simulink model "Part2"  (R2024b)
settings: Solver=ode4  StartTime=0.0  StopTime=T_SIM  FixedStep=T_s  RelTol=1e-3
values from neighbouring files (symbols this model uses):
  D = diag([0.001, 0.001, 0.0175/6, 0.0175/6, 0.0175/6, 0.0175/6*T_s, 0.0175/6*T_s].^2)    [P2_script.m]    (also in workspace_full.mat = [1e-06 0 0 0 0 0 0 0 1e-06 0 0 0 ... (49 elements, 7x7)])
  d_id = d_cal_hat    [P2_script.m]
  H = [H_motion_cap ; H_enc; H_gyro]    [P2_script.m]    (also in workspace_full.mat = [0 0 0 0 0 0 1 0 0 1 0 0 ... (14 elements, 2x7)])
  H_enc = [0, 0, 0, 1, 0, 0, 0 ... (first row only)    [P2_script.m]
  H_gyro = [0, 0, 0, 0, 0, -r_id/d_id, r_id/d_id]    [P2_script.m]
  H_motion_cap = [1, 0, 0, 0, 0, 0, 0 ... (first row only)    [P2_script.m]
  P_INIT_EKF = diag([0.001, 0.001, 0.0175/6, 0.0175/6, 0.0175/6, 0.0175/6*T_s, 0.0175/6*T_s].^2)    [P2_script.m]    (also in workspace_full.mat = [1e-06 0 0 0 0 0 0 0 1e-06 0 0 0 ... (49 elements, 7x7)])
  p_loss = p_loss_values(3)    [P2_script.m]
  PHI_INIT = [0;0]    [P2_script.m]    (also in workspace_full.mat = [0 0])
  Q_INIT_LOC = Q_INIT    [P2_script.m]    (also in workspace_full.mat = [0 0 0.463647609001])
  R_1 = diag([ENCODER_QUANTIZATION/6, ENCODER_QUANTIZATION/6].^2)    [P2_script.m]
  R_2 = diag(([ENCODER_QUANTIZATION/6, ENCODER_QUANTIZATION/6, var_IMU]).^2)    [P2_script.m]    (also in workspace_full.mat = [6.53638071556e-08  0; 0  6.53638071556e-08])
  R_3 = diag(([var_motion_capture, var_motion_capture, var_motion_capture,               ENCODER_QUANTIZATION/6, ENCODER_QUANTIZATION/6, var_IMU]).^2)    [P2_script.m]    (also in workspace_full.mat = [1e-06  0  0; 0  6.53638071556e-08  0; 0  0  6.53638071556e-)
  r_id = r_cal_hat    [P2_script.m]
  T_s = 0.04    [P2_script.m]    (also in workspace_full.mat)
  test_case = 3    [P2_script.m]
  Z_INIT_EKF = [Q_INIT; 0; 0; 0; 0]    [P2_script.m]    (also in workspace_full.mat = [0 0 0.463647609001 0 0 0 0])
settings Model: Creator=tomailoren  LastModifiedBy=loren
settings OptimizationCC: DefaultParameterBehavior=Inlined  EnhancedBackFolding=on  PassReuseOutputArgsAs=Individual arguments  ZeroExternalMemoryAtStartup=off  ZeroInternalMemoryAtStartup=off  MaxStackSize=64  OptimizeBlockOrder=speed  DifferentSizesBufferReuse=on  OptimizationCustomize=off  EfficientTunableParamExpr=on
settings DebuggingCC: ParameterTunabilityLossMsg=error
settings HardwareCC: ProdBitPerPointer=32  ProdBitPerSizeT=32  ProdBitPerPtrDiffT=32  ProdLargestAtomicFloat=None  ProdIntDivRoundTo=Undefined  ProdEndianess=Unspecified  ProdWordSize=32  ProdHWDeviceType=Generic->Unspecified (assume 32-bit Generic)
settings SFSimCC: MATLABDynamicMemAlloc=off
settings RTWCC: Description=Embedded Coder  SystemTargetFile=ert.tlc  HardwareBoard=Robot Operating System (ROS)  TLCOptions="-aInlineSetEventsForThisBaseRateFcn=TLC_FALSE -aSuppressMultiTaskScheduler=TLC_FALSE  -aRateBasedStepFcn=0"  TemplateMakefile=ert_default_tmf  Toolchain=Catkin  TargetLang=C++
settings CodeAppCC: ForceParamTrailComments=on  IgnoreCustomStorageClasses=off  OperatorAnnotations=on  SimulinkDataObjDesc=on  SFDataObjDesc=on  InsertBlockDesc=on

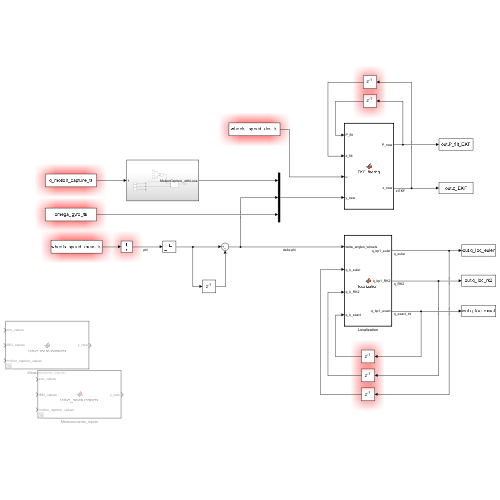
[thumbnail: Simulink's stored preview of the top-level diagram]
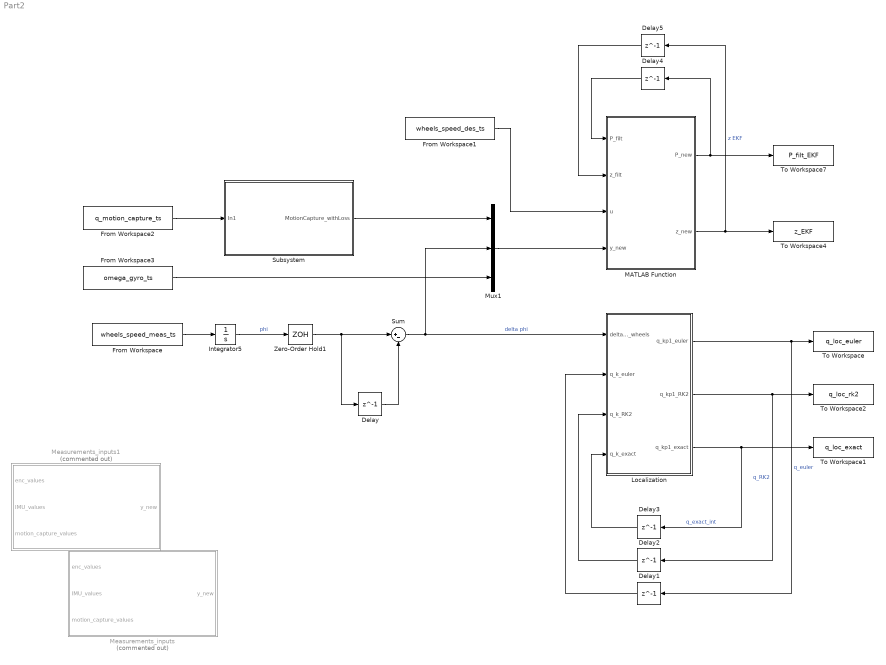
== system Part2 ==
  Delay : Delay  DelayLength=1  InitialCondition=[0;0]  SampleTime=T_s
  Delay1 : Delay  DelayLength=1  InitialCondition=Q_INIT_LOC
  Delay2 : Delay  DelayLength=1  InitialCondition=Q_INIT_LOC
  Delay3 : Delay  DelayLength=1  InitialCondition=Q_INIT_LOC
  Delay4 : Delay  DelayLength=1  InitialCondition=P_INIT_EKF  SampleTime=T_s
  Delay5 : Delay  DelayLength=1  InitialCondition=Z_INIT_EKF  SampleTime=T_s
  From Workspace : FromWorkspace  VariableName=wheels_speed_meas_ts
  From Workspace1 : FromWorkspace  VariableName=wheels_speed_des_ts
  From Workspace2 : FromWorkspace  VariableName=q_motion_capture_ts
  From Workspace3 : FromWorkspace  VariableName=omega_gyro_ts
  Integrator5 : Integrator  InitialCondition=PHI_INIT
  Localization : MATLAB Function  TreatAsAtomicUnit=on
  MATLAB Function : MATLAB Function  TreatAsAtomicUnit=on
  Measurements_inputs : MATLAB Function  Commented=on  TreatAsAtomicUnit=on
  Measurements_inputs1 : MATLAB Function  Commented=on  TreatAsAtomicUnit=on
  Mux1 : Mux  Inputs=3
  Subsystem : Subsystem
  Sum : Sum  Inputs=|+-
  To Workspace : ToWorkspace  VariableName=q_loc_euler  SaveFormat=Structure With Time  SampleTime=-1
  To Workspace1 : ToWorkspace  VariableName=q_loc_exact  SaveFormat=Structure With Time  SampleTime=-1
  To Workspace2 : ToWorkspace  VariableName=q_loc_rk2  SaveFormat=Structure With Time  SampleTime=-1
  To Workspace4 : ToWorkspace  VariableName=z_EKF  SaveFormat=Structure With Time  SampleTime=-1
  To Workspace7 : ToWorkspace  VariableName=P_filt_EKF  SaveFormat=Structure With Time  SampleTime=-1
  Zero-Order Hold1 : ZeroOrderHold  SampleTime=T_s
  wires:
  MATLAB Function/2(z_new) -> Delay5/1, To Workspace4/1  "z EKF"
  Delay1/1 -> Localization/2(q_k_euler)
  Zero-Order Hold1/1 -> Delay/1, Sum/1
  Delay5/1 -> MATLAB Function/2(z_filt)
  Delay/1 -> Sum/2
  Delay3/1 -> Localization/4(q_k_exact)
  Integrator5/1 -> Zero-Order Hold1/1  "phi"
  Localization/2(q_kp1_RK2) -> To Workspace2/1, Delay2/1  "q_RK2"
  Localization/1(q_kp1_euler) -> To Workspace/1, Delay1/1  "q_euler"
  Delay2/1 -> Localization/3(q_k_RK2)
  Sum/1 -> Mux1/2, Localization/1(delta_angles_wheels)  "delta phi"
  Delay4/1 -> MATLAB Function/1(P_filt)
  Localization/3(q_kp1_exact) -> To Workspace1/1, Delay3/1  "q_exact_int"
  MATLAB Function/1(P_new) -> Delay4/1, To Workspace7/1
  From Workspace/1 -> Integrator5/1
  From Workspace1/1 -> MATLAB Function/3(u)
  Mux1/1 -> MATLAB Function/4(y_new)
  From Workspace3/1 -> Mux1/3
  From Workspace2/1 -> Subsystem/1(In1)
  Subsystem/1(MotionCapture_withLoss) -> Mux1/1

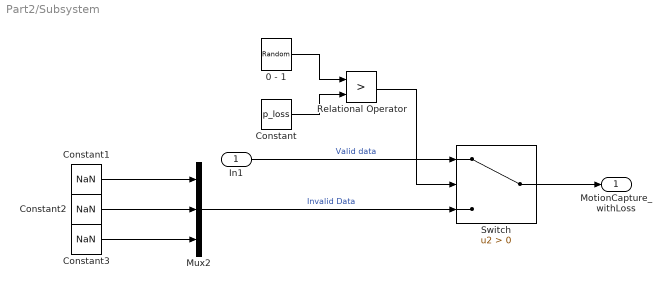
== system Part2/Subsystem ==
  In1 : Inport
  0 - 1 : UniformRandomNumber  Minimum=0  SampleTime=T_s
  Constant : Constant  Value=p_loss
  Constant1 : Constant  Value=NaN
  Constant2 : Constant  Value=NaN
  Constant3 : Constant  Value=NaN
  Mux2 : Mux  Inputs=3
  Relational Operator : RelationalOperator  Operator=>  OutDataTypeStr=boolean  RndMeth=Simplest  InputSameDT=off
  Switch : Switch  Criteria=u2 > Threshold  SaturateOnIntegerOverflow=off  InputSameDT=off
  MotionCapture_withLoss : Outport
  wires:
  0 - 1/1 -> Relational Operator/1
  Constant/1 -> Relational Operator/2
  Switch/1 -> MotionCapture_withLoss/1
  Relational Operator/1 -> Switch/2
  Constant2/1 -> Mux2/2
  Mux2/1 -> Switch/3  "Invalid Data"
  Constant1/1 -> Mux2/1
  In1/1 -> Switch/1  "Valid data"
  Constant3/1 -> Mux2/3

== matlab function Part2/Measurements_inputs1 ==
  data: enc_values input; y_new output; IMU_values input; motion_capture_values input; test_case parameter
function y_new = select_measurements(enc_values, IMU_values, motion_capture_values, test_case)
   
    % enc_values (delta_phi)
    % IMU_values (w_gyro)
    % Motion_capture (state q)

    y_new = zeros(6, 1);
    % y_new = [x; y; theta; delta_phi_L; delta_phi_R; omega_gyro]
    
    if test_case == 1
        % Test 1: Only Encoder
        y_new(4) = enc_values(1);
        y_new(5) = enc_values(2);
        
    elseif test_case == 2
        % Test 2: Encoder + IMU
        y_new(4) = enc_values(1);
        y_new(5) = enc_values(2);
        y_new(6) = IMU_values(1);
        
    elseif test_case == 3
        % Test 3: Encoder + IMU + Motion Capture
        y_new(1) = motion_capture_values(1);
        y_new(2) = motion_capture_values(2);
        y_new(3) = motion_capture_values(3);
        y_new(4) = enc_values(1);
        y_new(5) = enc_values(2);
        y_new(6) = IMU_values(1);
    end
end

== matlab function Part2/Measurements_inputs ==
  data: enc_values input; y_new output; IMU_values input; motion_capture_values input; test_case parameter
function y_new = select_measurements(enc_values, IMU_values, motion_capture_values, test_case)
   
    % enc_values (delta_phi)
    % IMU_values (w_gyro)
    % Motion_capture (state q)

    % y_new = [x; y; theta; delta_phi_L; delta_phi_R; omega_gyro]
    y_new = zeros(1,6);

    if test_case == 1
        % Test 1: Only Encoder
        y_new(1) = enc_values(1);
        y_new(2) = enc_values(2);
        
    elseif test_case == 2
        % Test 2: Encoder + IMU
        y_new(1) = enc_values(1);
        y_new(2) = enc_values(2);
        y_new(3) = IMU_values(1);
        
    elseif test_case == 3
        % Test 3: Encoder + IMU + Motion Capture        
        y_new(1) = motion_capture_values(1);
        y_new(2) = motion_capture_values(2);
        y_new(3) = motion_capture_values(3);
        y_new(4) = enc_values(1);
        y_new(5) = enc_values(2);
        y_new(6) = IMU_values(1);
    end
    
end

== matlab function Part2/Localization ==
  data: delta_angles_wheels input; q_k_euler input; q_k_RK2 input; q_k_exact input; r_id parameter; d_id parameter; q_kp1_euler output; T_s parameter; q_kp1_RK2 output; q_kp1_exact output
function [q_kp1_euler, q_kp1_RK2, q_kp1_exact] = localization(delta_angles_wheels, q_k_euler, q_k_RK2, q_k_exact, r_id, d_id, T_s)

    r = r_id;
    d = d_id;

    % extraction data
    delta_phi_L = delta_angles_wheels(1);
    delta_phi_R = delta_angles_wheels(2);

    x_k_euler = q_k_euler(1); 
    y_k_euler = q_k_euler(2); 
    theta_k_euler = q_k_euler(3);
    
    x_k_RK2 = q_k_RK2(1); 
    y_k_RK2 = q_k_RK2(2); 
    theta_k_RK2 = q_k_RK2(3);

    x_k_exact = q_k_exact(1);
    y_k_exact = q_k_exact(2); 
    theta_k_exact = q_k_exact(3);


    % velocities estimate
    v_k = r / (2*T_s) * (delta_phi_R + delta_phi_L);
    w_k = r / (d*T_s) * (delta_phi_R - delta_phi_L);
    
    % Euler integration
    x_kp1_euler = x_k_euler + v_k * T_s * cos(theta_k_euler);
    y_kp1_euler = y_k_euler + v_k * T_s * sin(theta_k_euler);
    theta_kp1_euler = theta_k_euler + w_k * T_s;
    
    q_kp1_euler = [x_kp1_euler; y_kp1_euler; theta_kp1_euler];
    
    % RK2 Integration
    x_kp1_RK2 = x_k_RK2 + v_k * T_s * cos(theta_k_RK2 + (w_k * T_s)/2);
    y_kp1_RK2 = y_k_RK2 + v_k * T_s * sin(theta_k_RK2 + (w_k * T_s)/2);
    theta_kp1_RK2 = theta_k_RK2 + w_k * T_s;
    
    q_kp1_RK2 = [x_kp1_RK2; y_kp1_RK2; theta_kp1_RK2];
    
    % Exact Integration
    if abs(w_k) < 1e-4
        % use RK2 approximation to avoid division by zero when w_k is near 0
        x_kp1_exact = x_k_exact + v_k * T_s * cos(theta_k_exact + (w_k * T_s)/2);
        y_kp1_exact = y_k_exact + v_k * T_s * sin(theta_k_exact + (w_k * T_s)/2);
    else
        % Exact formulas
        x_kp1_exact = x_k_exact + (v_k / w_k) * (sin(theta_k_exact + w_k * T_s) - sin(theta_k_exact));
        y_kp1_exact = y_k_exact - (v_k / w_k) * (cos(theta_k_exact + w_k * T_s) - cos(theta_k_exact));
    end
    theta_kp1_exact = theta_k_exact + w_k * T_s;
    
    q_kp1_exact = [x_kp1_exact; y_kp1_exact; theta_kp1_exact];
    
end

== matlab function Part2/MATLAB Function ==
  data: P_filt input; P_new output; z_filt input; z_new output; u input; y_new input; D parameter; R_1 parameter; H parameter; T_s parameter; r_id parameter; d_id parameter; test_case parameter; H_enc parameter; H_gyro parameter; H_motion_cap parameter; R_2 parameter; R_3 parameter
function [P_new, z_new] = EKF_filtering(P_filt, z_filt, u, y_new, D, R_1, H, T_s, r_id, d_id, test_case, H_enc, H_gyro, H_motion_cap, R_2, R_3)

    % Def state z_filt: [xk , yk , thetak , delta_phi_L_km1 , delta_phi_R_km1 , wLk , wRk ]

    r = r_id;
    d = d_id;
        
    % Extraction variables
    x_k = z_filt(1);
    y_k = z_filt(2);
    theta_k = z_filt(3);
    delta_phi_L_km1 = z_filt(4);
    delta_phi_R_km1 = z_filt(5); 
    wL_k = z_filt(6);               % estimate wheels velocities
    wR_k = z_filt(7);
    
    uL_k = u(1);                    % actual wheels velocities (from command input v,w)
    uR_k = u(2);

    % ----------------------

    % PREDICT STEP
    v_k = (r/2) * (wL_k + wR_k);
    omega_k = (r/d) * (wR_k - wL_k);
    theta_mean = theta_k + (omega_k * T_s) / 2;
        
    % State Prediction (approximation with RK2)
    x_kp1 = x_k + v_k * T_s * cos(theta_mean);
    y_kp1 = y_k + v_k * T_s * sin(theta_mean);
    theta_kp1 = theta_k + omega_k * T_s;
    
    delta_phi_L_k = wL_k * T_s;
    delta_phi_R_k = wR_k * T_s;
    
    wL_kp1 = uL_k; 
    wR_kp1 = uR_k;
    
    z_hat = [x_kp1; y_kp1; theta_kp1; delta_phi_L_k; delta_phi_R_k; wL_kp1; wR_kp1];
    
    % F derivation
    F = zeros(7,7);
    
    F(1,1) = 1;
    F(1, 3) = -T_s * v_k * sin(theta_mean);
    F(1, 6) = (T_s * r / 2) * cos(theta_mean) - v_k * T_s * sin(theta_mean) * (-T_s * r / (2 * d));
    F(1, 7) = (T_s * r / 2) * cos(theta_mean) - v_k * T_s * sin(theta_mean) * (T_s * r / (2 * d));
    
    F(2,2) = 1;
    F(2, 3) = v_k * T_s * cos(theta_mean);
    F(2, 6) = (T_s * r / 2) * sin(theta_mean) + v_k * T_s * cos(theta_mean) * (-T_s * r / (2 * d));
    F(2, 7) = (T_s * r / 2) * sin(theta_mean) + v_k * T_s * cos(theta_mean) * (T_s * r / (2 * d));

    F(3,3) = 1;
    F(3, 6) = -T_s * r / d;
    F(3, 7) = T_s * r / d;

    F(4, 6) = T_s;
    F(5, 7) = T_s;
    
    % Covariance Prediction
    P_hat = F * P_filt * F' + D;
    
    % ----------------------

    % UPDATE STEP
    % H and R will depend on the measurement data y_new and Test_case

    % enc_values (delta_phi)
    % IMU_values (w_gyro)
    % Motion_capture (state q)

    % y_new = [x; y; theta; delta_phi_L; delta_phi_R; omega_gyro]

    %% OBSERVATION MATRIX H ALWAYS FULL (6X7) AND ALSO Y_NEW (6X1) 
    H_full = [H_motion_cap; H_enc; H_gyro];
    y_meas = y_new; 
    
    % Usiamo la R_3 (6x6) come base
    R_current = R_3;
    INFINITY_VAR = 1e9; % Incertezza "infinita" per spegnere il Kalman Gain
    
    if test_case == 1
        % TEST 1: Mocap (1:3) e Gyro (6) spenti
        y_meas(1:3) = 0;  % <--- FORZIAMO A ZERO COME HAI INTUITO
        y_meas(6)   = 0;  % <--- FORZIAMO A ZERO
        
        R_current(1,1) = INFINITY_VAR; R_current(2,2) = INFINITY_VAR; R_current(3,3) = INFINITY_VAR;
        R_current(6,6) = INFINITY_VAR;
        
    elseif test_case == 2
        % TEST 2: Solo Mocap (1:3) spento
        y_meas(1:3) = 0;  % <--- FORZIAMO A ZERO
        
        R_current(1,1) = INFINITY_VAR; R_current(2,2) = INFINITY_VAR; R_current(3,3) = INFINITY_VAR;
        
    elseif test_case == 3
        % TEST 3: Tutti attivi, perdita pacchetto Mocap dinamica
        if any(isnan(y_new(1:3)))
            y_meas(1:3) = 0; % Mocap perso -> forziamo a zero
            R_current(1,1) = INFINITY_VAR; R_current(2,2) = INFINITY_VAR; R_current(3,3) = INFINITY_VAR;
        end
    end
    
    % Innovation e_pred
    y_hat = H_full * z_hat;
    e_kp1 = y_meas - y_hat;
    
    % Kalman Gain K_pred
    K = P_hat * H_full' / (H_full * P_hat * H_full' + R_current);   
    
    % State and Covariance Update
    z_new = z_hat + K * e_kp1;
    P_new = P_hat - K * H_full * P_hat;


%% IT CRUSH BECAUSE OF CHANGE OF MATRIX DURING SIMULATION
%     if test_case == 1
%         % Test 1: Only Encoder
%         y_meas = y_new(4:5);
%         H = H_enc;
%         R = R_1;
% 
%     elseif test_case == 2
%         % Test 2: Encoder + IMU
%         y_meas = y_new(4:6);
%         H = [H_enc; H_gyro];
%         R = R_2;
% 
%     elseif test_case == 3
%         % Test 3: Encoder + IMU + Motion Capture        
%         if any(isnan(y_new(1:3)))
%             % Motion Capture data lost --> Downgrade to ENC + IMU
%             y_meas = y_new(4:6);
%             H = [H_enc; H_gyro];
%             R = R_2;
%         else
%             % All sensors available
%             y_meas = y_new;
%             H = [H_motion_cap; H_enc; H_gyro];
%             R = R_3;
%         end
%     end
% 
% 
%     % Innovation e_pred
%     y_hat = H * z_hat;
%     e_kp1 = y_meas - y_hat;
% 
%     % Kalman Gain K_pred
%     K = P_hat * H' / ( H * P_hat * H' + R);   
% 
%     % State and Covariance Update
%     z_new = z_hat + K * e_kp1;
%     P_new = P_hat - K * H * P_hat;
% 
end
